simulink model "verify_EnergyMeter_mdl"  (R2016b)
settings: Solver=ode45  StartTime=0.0  StopTime=3600  MaxStep=100  RelTol=1e-3  EnableMultiTasking=on
libraries: carnot x3
settings Model: Creator=drhf  LastModifiedBy=drhf
settings DataIOCC: SaveFormat=Array  SignalLoggingSaveFormat=ModelDataLogs
settings OptimizationCC: ExpressionDepthLimit=2147483647  LifeSpan=inf
settings DebuggingCC: UnderspecifiedInitializationDetection=Classic  MergeDetectMultiDrivingBlocksExec=none  SolverPrmCheckMsg=warning  FcnCallInpInsideContextMsg=warning  StateNameClashWarn=warning  SFUnexpectedBacktrackingDiag=warning  SFNoUnconditionalDefaultTransitionDiag=warning  SFExecutionAtInitializationDiag=none
settings HardwareCC: ProdBitPerPointer=32  ProdBitPerSizeT=32  ProdBitPerPtrDiffT=32  ProdLargestAtomicFloat=None  ProdIntDivRoundTo=Undefined  ProdEndianess=Unspecified  ProdWordSize=32  ProdHWDeviceType=32-bit Generic
settings ModelReferenceCC: PropagateSignalLabelsOutOfModel=off
settings GRTTargetCC: TargetLangStandard=C89/C90 (ANSI)  GeneratePreprocessorConditionals=Disable all  CombineOutputUpdateFcns=off  GRTInterface=on
settings ConfigComp: CovMetricSettings=dw  CovHtmlReporting=on  CovSaveCumulativeToWorkspaceVar=on  CovSaveSingleToWorkspaceVar=on  CovExternalEMLEnable=off

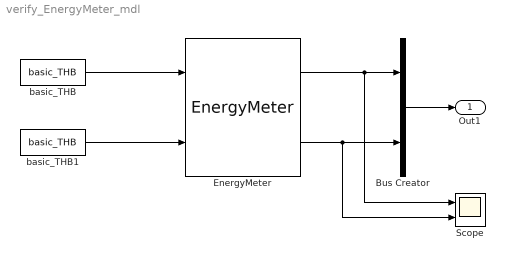
== system verify_EnergyMeter_mdl ==
  Bus Creator : BusCreator  Inputs=2
  EnergyMeter : carnot/Control/EnergyMeter
  Scope : Scope  NumInputPorts=2
  basic_THB : carnot/Basic/Hydraulics/basic_THB  t=70  mdot=200/3600  p=1e5  ID=Pressure Drop from Massflow  fluid=Water  mix=0  mix2=0  mix3=0  dia=0.02  hgt=0
  basic_THB1 : carnot/Basic/Hydraulics/basic_THB  t=50  mdot=200/3600  p=1e5  ID=Pressure Drop from Massflow  fluid=Water  mix=0  mix2=0  mix3=0  dia=0.02  hgt=0
  Out1 : Outport
  wires:
  Bus Creator/1 -> Out1/1
  basic_THB/1 -> EnergyMeter/1
  basic_THB1/1 -> EnergyMeter/2
  EnergyMeter/1 -> Scope/1, Bus Creator/1
  EnergyMeter/2 -> Scope/2, Bus Creator/2
